simulink model "RobotSimulation1"  (R2020b)
settings: Solver=ode45  StartTime=0.0  StopTime=2  MaxStep=1e-6  RelTol=1e-3%1e-10
model workspace (MAT data in the model file):
  H = 0.2
  L = 0.1
  Mchoice = 1
  q0 = [-1.31838984174e-15; -0.785398163397; 0.0707106781187]
  qdot0 = [0; 0; 0]
settings Model: OrderedModelArguments=off  Creator=alons  LastModifiedBy=שחר צדוק
settings SolverCC: ConsecutiveZCsStepRelTol=eps%10*128*eps

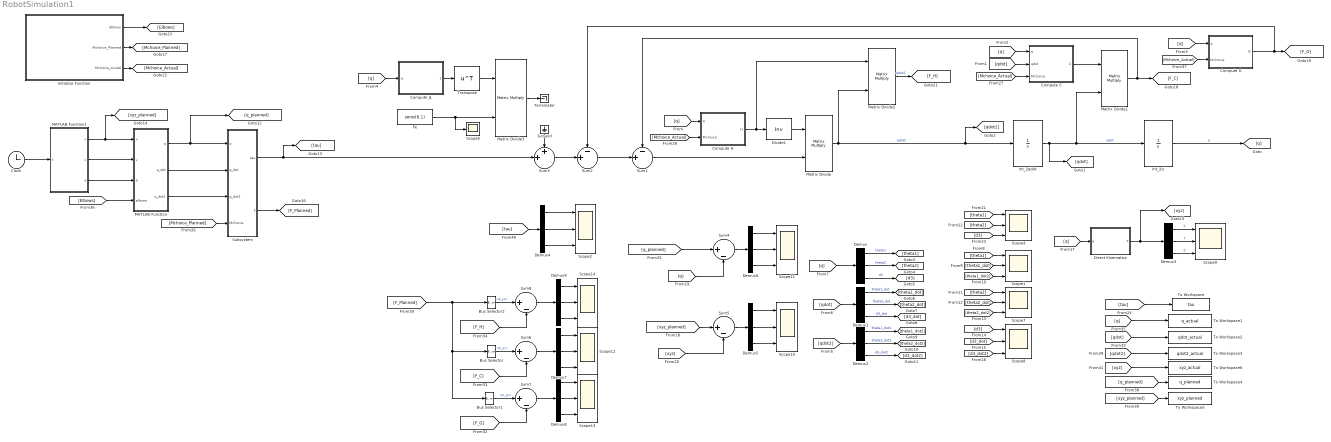
== system RobotSimulation1 ==
  Bus Selector : BusSelector  OutputSignals=F_C
  Bus Selector1 : BusSelector  OutputSignals=F_G
  Bus Selector2 : BusSelector  OutputSignals=F_H
  Clock : Clock
  Compute C : MATLAB Function  TreatAsAtomicUnit=on
  Compute G : MATLAB Function  TreatAsAtomicUnit=on
  Compute H : MATLAB Function  TreatAsAtomicUnit=on
  Compute JL : MATLAB Function  TreatAsAtomicUnit=on
  Demux{,1..9} (10 alike) : Demux  Outputs=3
  Direct Kinematics : MATLAB Function  TreatAsAtomicUnit=on
  Divide1 : Product  Inputs=/  Multiplication=Matrix(*)
  Fe : Constant  Value=zeros(6,1)
  Ground : Ground
  Initialize Function : Subsystem  TreatAsAtomicUnit=on
  Int_2q : Integrator  InitialCondition=[0,0,0]'
  Int_2qdot : Integrator  InitialCondition=[0,0,0]'
  MATLAB Function : MATLAB Function  TreatAsAtomicUnit=on
  MATLAB Function1 : MATLAB Function  TreatAsAtomicUnit=on
  Matrix Divide{,1..3} (4 alike) : Product  Inputs=**  Multiplication=Matrix(*)
  Scope{1..2,4,7..14} (11 alike) : Scope  NumInputPorts=3
  Scope5 : Scope
  Subsystem : Subsystem
  Sum1 : Sum  Inputs=-+|
  Sum2 : Sum  Inputs=-+|
  Sum3 : Sum  Inputs=++|
  Sum{4..8} (5 alike) : Sum  Inputs=|+-
  Terminator : Terminator
  To Workspace : ToWorkspace  VariableName=tau  SaveFormat=Timeseries  SampleTime=-1
  To Workspace1 : ToWorkspace  VariableName=q_actual  SaveFormat=Timeseries  SampleTime=-1
  To Workspace2 : ToWorkspace  VariableName=qdot_actual  SaveFormat=Timeseries  SampleTime=-1
  To Workspace3 : ToWorkspace  VariableName=qdot2_actual  SaveFormat=Timeseries  SampleTime=-1
  To Workspace4 : ToWorkspace  VariableName=q_planned  SaveFormat=Timeseries  SampleTime=-1
  To Workspace5 : ToWorkspace  VariableName=xyz_planned  SaveFormat=Timeseries  SampleTime=-1
  To Workspace6 : ToWorkspace  VariableName=xyz_actual  SaveFormat=Timeseries  SampleTime=-1
  Transpose : Math  Operator=transpose  SaturateOnIntegerOverflow=on
  wires:
  Compute H/1(H) -> Matrix Divide2/1, Divide1/1
  Compute C/1(C) -> Matrix Divide1/1
  Int_2qdot/1 -> [qdot], Matrix Divide1/2, Int_2q/1  "qdot"
  Int_2q/1 -> [q]  "q"
  Divide1/1 -> Matrix Divide/1
  Matrix Divide/1 -> Matrix Divide2/2, [qdot2], Int_2qdot/1  "qdot2"
  Sum2/1 -> Sum1/2
  Sum1/1 -> Matrix Divide/2
  Compute G/1(G) -> [F_G], Sum2/1
  Sum3/1 -> Sum2/2
  Compute JL/1(J) -> Transpose/1
  Transpose/1 -> Matrix Divide3/1
  Fe/1 -> Scope5/1, Matrix Divide3/2
  [q] -> Compute H/1(q)
  [qdot] -> Compute C/2(qdot)
  [q] -> Compute C/1(q)
  [q] -> Compute G/1(q)
  Matrix Divide1/1 -> [F_C], Sum1/1
  [q] -> Compute JL/1(q)
  [Mchoice_Actual] -> Compute C/3(Mchoice)
  [Mchoice_Actual] -> Compute G/2(Mchoice)
  [Mchoice_Actual] -> Compute H/2(Mchoice)
  Subsystem/1(tau) -> [tau], Sum3/2
  [q] -> Demux/1
  [qdot] -> Demux1/1
  [qdot2] -> Demux2/1
  Demux/1 -> [theta1]  "theta1"
  Demux1/1 -> [theta1_dot]  "theta1_dot"
  Demux/3 -> [d3]  "d3"
  Demux/2 -> [theta2]  "theta2"
  Demux1/2 -> [theta2_dot]  "theta2_dot"
  Demux1/3 -> [d3_dot]  "d3_dot"
  Demux2/1 -> [theta1_dot2]  "theta1_dot2"
  Demux2/2 -> [theta2_dot2]  "theta2_dot2"
  Demux2/3 -> [d3_dot2]  "d3_dot2"
  [theta1] -> Scope1/1
  [theta1_dot] -> Scope1/2
  [theta1_dot2] -> Scope1/3
  [theta2] -> Scope7/1
  [theta2_dot] -> Scope7/2
  [theta2_dot2] -> Scope7/3
  [d3] -> Scope8/1
  [d3_dot] -> Scope8/2
  [d3_dot2] -> Scope8/3
  [q] -> Direct Kinematics/1(q)
  Direct Kinematics/1(T) -> [xyz], Demux3/1
  Demux3/1 -> Scope9/1  "X"
  Demux3/2 -> Scope9/2  "Y"
  Demux3/3 -> Scope9/3  "Z"
  Demux4/1 -> Scope2/1
  Demux4/2 -> Scope2/2
  Demux4/3 -> Scope2/3
  Clock/1 -> MATLAB Function1/1(t)
  MATLAB Function1/1(x) -> [xyz_planned], MATLAB Function/1(x)
  MATLAB Function1/2(v) -> MATLAB Function/2(v)
  MATLAB Function1/3(a) -> MATLAB Function/3(a)
  [Elbows] -> MATLAB Function/4(elbows)
  MATLAB Function/2(q_dot) -> Subsystem/2(q_dot)
  MATLAB Function/3(q_dot2) -> Subsystem/3(q_dot2)
  MATLAB Function/1(q) -> [q_planned], Subsystem/1(q)
  [theta1] -> Scope4/1
  [theta2] -> Scope4/2
  [d3] -> Scope4/3
  [q_planned] -> Sum4/1
  [q] -> Sum4/2
  [xyz_planned] -> Sum5/1
  [xyz] -> Sum5/2
  Sum5/1 -> Demux5/1
  Demux5/1 -> Scope10/1
  Demux5/2 -> Scope10/2
  Demux5/3 -> Scope10/3
  Demux6/1 -> Scope11/1
  Demux6/2 -> Scope11/2
  Sum4/1 -> Demux6/1
  Demux6/3 -> Scope11/3
  [tau] -> To Workspace/1
  Subsystem/2(F) -> [F_Planned]
  [Mchoice_Planned] -> Subsystem/4(Mchoice)
  Bus Selector/1 -> Sum6/1  "<F_C>"
  [F_C] -> Sum6/2
  Sum6/1 -> Demux7/1
  Demux7/1 -> Scope12/1
  Demux7/2 -> Scope12/2
  Demux7/3 -> Scope12/3
  Bus Selector1/1 -> Sum7/1  "<F_G>"
  [F_G] -> Sum7/2
  Demux8/1 -> Scope13/1
  Demux8/2 -> Scope13/2
  Demux8/3 -> Scope13/3
  Sum7/1 -> Demux8/1
  Demux9/2 -> Scope14/2
  [F_H] -> Sum8/2
  Sum8/1 -> Demux9/1
  Demux9/3 -> Scope14/3
  Demux9/1 -> Scope14/1
  Bus Selector2/1 -> Sum8/1  "<F_H>"
  [F_Planned] -> Bus Selector1/1, Bus Selector/1, Bus Selector2/1
  Matrix Divide2/1 -> [F_H]  "qdot2"
  Initialize Function/2(Mchoice_Planned) -> [Mchoice_Planned]
  Initialize Function/1(Elbows) -> [Elbows]
  Matrix Divide3/1 -> Terminator/1
  Ground/1 -> Sum3/1
  Initialize Function/3(Mchoice_Acutal) -> [Mchoice_Actual]
  [q] -> To Workspace1/1
  [qdot] -> To Workspace2/1
  [qdot2] -> To Workspace3/1
  [xyz_planned] -> To Workspace5/1
  [q_planned] -> To Workspace4/1
  [tau] -> Demux4/1
  [xyz] -> To Workspace6/1

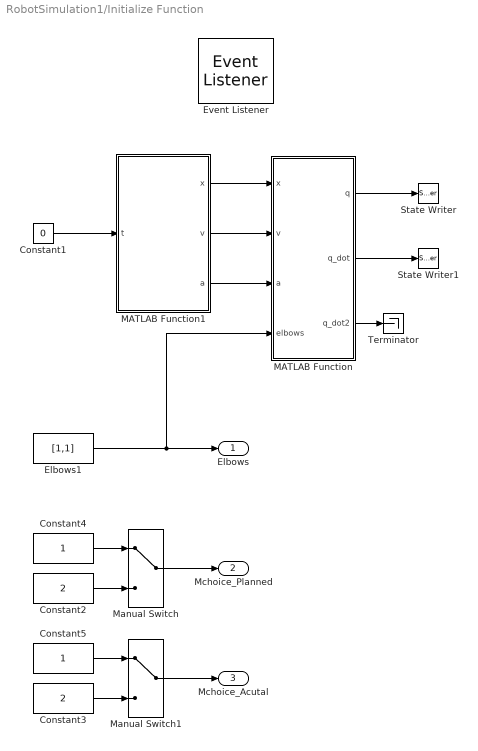
== system RobotSimulation1/Initialize Function ==
  Constant1 : Constant  Value=0
  Constant2 : Constant  Value=2
  Constant3 : Constant  Value=2
  Constant4 : Constant
  Constant5 : Constant
  Elbows1 : Constant  Value=[1,1]
  Event Listener : EventListener  DisableCoverage=on  EventName=reset
  MATLAB Function : MATLAB Function  TreatAsAtomicUnit=on
  MATLAB Function1 : MATLAB Function  TreatAsAtomicUnit=on
  Manual Switch : ManualSwitch
  Manual Switch1 : ManualSwitch
  State Writer : StateWriter  StateOwnerBlock=../../Int_2q
  State Writer1 : StateWriter  StateOwnerBlock=../../Int_2qdot
  Terminator : Terminator
  Elbows : Outport
  Mchoice_Planned : Outport  Port=2
  Mchoice_Acutal : Outport  Port=3
  wires:
  Constant1/1 -> MATLAB Function1/1(t)
  MATLAB Function1/1(x) -> MATLAB Function/1(x)
  MATLAB Function1/2(v) -> MATLAB Function/2(v)
  MATLAB Function1/3(a) -> MATLAB Function/3(a)
  Elbows1/1 -> Elbows/1, MATLAB Function/4(elbows)
  MATLAB Function/1(q) -> State Writer/1
  MATLAB Function/2(q_dot) -> State Writer1/1
  MATLAB Function/3(q_dot2) -> Terminator/1
  Constant4/1 -> Manual Switch/1
  Constant2/1 -> Manual Switch/2
  Manual Switch/1 -> Mchoice_Planned/1
  Constant3/1 -> Manual Switch1/2
  Constant5/1 -> Manual Switch1/1
  Manual Switch1/1 -> Mchoice_Acutal/1

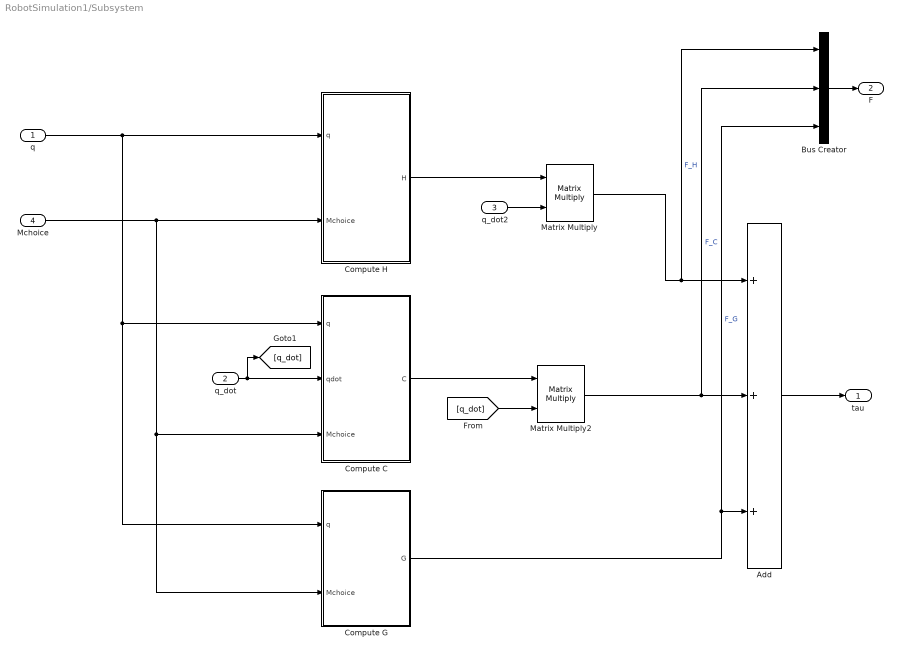
== system RobotSimulation1/Subsystem ==
  q : Inport
  q_dot : Inport  Port=2
  q_dot2 : Inport  Port=3
  Mchoice : Inport  Port=4
  Add : Sum  Inputs=+++
  Bus Creator : BusCreator  Inputs=3
  Compute C : MATLAB Function  TreatAsAtomicUnit=on
  Compute G : MATLAB Function  TreatAsAtomicUnit=on
  Compute H : MATLAB Function  TreatAsAtomicUnit=on
  Matrix Multiply : Product  Multiplication=Matrix(*)
  Matrix Multiply2 : Product  Multiplication=Matrix(*)
  tau : Outport
  F : Outport  Port=2
  wires:
  Compute H/1(H) -> Matrix Multiply/1
  Compute C/1(C) -> Matrix Multiply2/1
  q/1 -> Compute H/1(q), Compute G/1(q), Compute C/1(q)
  q_dot/1 -> Compute C/2(qdot), [q_dot]
  q_dot2/1 -> Matrix Multiply/2
  [q_dot] -> Matrix Multiply2/2
  Matrix Multiply/1 -> Bus Creator/1, Add/1  "F_H"
  Add/1 -> tau/1
  Bus Creator/1 -> F/1
  Matrix Multiply2/1 -> Bus Creator/2, Add/2  "F_C"
  Compute G/1(G) -> Bus Creator/3, Add/3  "F_G"
  Mchoice/1 -> Compute H/2(Mchoice), Compute G/2(Mchoice), Compute C/3(Mchoice)

== matlab function RobotSimulation1/Subsystem/Compute G ==
  data: q input; G output; Mchoice input
function G = ComputeG(q,Mchoice)
f_GdynM1=@(in1)[0.0;sin(in1(2,:)).*(in1(3,:).*1.0e+1-pi.*4.3875e-2+in1(3,:).*pi.*(3.51e+2./4.0e+2)).*(-4.905e-1);cos(in1(2,:)).*(pi.*4.3875e-2+1.0./2.0).*(9.81e+2./1.0e+2)];
f_GdynM2=@(in1)[0.0;sin(in1(2,:)).*(in1(3,:).*1.2e+1-pi.*4.3875e-2+in1(3,:).*pi.*(3.51e+2./4.0e+2)).*(-4.905e-1);cos(in1(2,:)).*(pi.*4.3875e-2+3.0./5.0).*(9.81e+2./1.0e+2)];
if Mchoice==1
    G=f_GdynM1(q);
else %==2
    G=f_GdynM2(q);
end
end

== matlab function RobotSimulation1/Subsystem/Compute H ==
  data: q input; H output; Mchoice input
function H = ComputeH(q,Mchoice)
f_HdynM1=@(in1)reshape([pi.*5.85e-4+(in1(3,:).^2.*sin(in1(2,:)).^2)./2.0+pi.*sin(in1(2,:)).^2.*1.4625e-4-in1(3,:).*pi.*sin(in1(2,:)).^2.*4.3875e-3+in1(3,:).^2.*pi.*sin(in1(2,:)).^2.*4.3875e-2+1.0./2.0e+2,cos(in1(2,:)).*(in1(3,:).*1.0e+1-pi.*4.3875e-2+in1(3,:).*pi.*(3.51e+2./4.0e+2)).*(-1.0./2.0e+2),sin(in1(2,:)).*(pi.*4.3875e-2+1.0./2.0).*(-1.0./1.0e+1),cos(in1(2,:)).*(in1(3,:).*1.0e+1-pi.*4.3875e-2+in1(3,:).*pi.*(3.51e+2./4.0e+2)).*(-1.0./2.0e+2),pi.*3.65625e-5+in1(3,:).^2./2.0+pi.*(in1(3,:)-1.0./2.0e+1).^2.*4.3875e-2,0.0,sin(in1(2,:)).*(pi.*4.3875e-2+1.0./2.0).*(-1.0./1.0e+1),0.0,pi.*4.3875e-2+1.0./2.0],[3,3]);
f_HdynM2=@(in1)reshape([pi.*5.85e-4+in1(3,:).^2.*sin(in1(2,:)).^2.*(3.0./5.0)+pi.*sin(in1(2,:)).^2.*1.4625e-4-in1(3,:).*pi.*sin(in1(2,:)).^2.*4.3875e-3+in1(3,:).^2.*pi.*sin(in1(2,:)).^2.*4.3875e-2+3.0./5.0e+2,cos(in1(2,:)).*(in1(3,:).*1.2e+1-pi.*4.3875e-2+in1(3,:).*pi.*(3.51e+2./4.0e+2)).*(-1.0./2.0e+2),sin(in1(2,:)).*(pi.*4.3875e-2+3.0./5.0).*(-1.0./1.0e+1),cos(in1(2,:)).*(in1(3,:).*1.2e+1-pi.*4.3875e-2+in1(3,:).*pi.*(3.51e+2./4.0e+2)).*(-1.0./2.0e+2),pi.*3.65625e-5+in1(3,:).^2.*(3.0./5.0)+pi.*(in1(3,:)-1.0./2.0e+1).^2.*4.3875e-2,0.0,sin(in1(2,:)).*(pi.*4.3875e-2+3.0./5.0).*(-1.0./1.0e+1),0.0,pi.*4.3875e-2+3.0./5.0],[3,3]);
if Mchoice==1
    H=f_HdynM1(q);
else %==2
    H=f_HdynM2(q);
end

== matlab function RobotSimulation1/Compute C ==
  data: q input; C output; qdot input; Mchoice input
function C = ComputeC(q,qdot,Mchoice)
f_CdynM1=@(in1)reshape([in1(6,:).*((in1(3,:).*sin(in1(2,:)).^2)./2.0-pi.*sin(in1(2,:)).^2.*2.19375e-3+in1(3,:).*pi.*sin(in1(2,:)).^2.*4.3875e-2)+in1(5,:).*((in1(3,:).^2.*sin(in1(2,:).*2.0))./4.0+pi.*sin(in1(2,:).*2.0).*7.3125e-5-in1(3,:).*pi.*sin(in1(2,:).*2.0).*2.19375e-3+in1(3,:).^2.*pi.*sin(in1(2,:).*2.0).*2.19375e-2),in1(4,:).*sin(in1(2,:).*2.0).*(pi.*1.755e-1-in1(3,:).*pi.*5.265+in1(3,:).^2.*pi.*5.265e+1+in1(3,:).^2.*6.0e+2).*(-4.166666666666667e-4),in1(4,:).*sin(in1(2,:)).^2.*(in1(3,:).*1.0e+1-pi.*4.3875e-2+in1(3,:).*pi.*(3.51e+2./4.0e+2)).*(-1.0./2.0e+1),in1(4,:).*((in1(3,:).^2.*sin(in1(2,:).*2.0))./4.0+pi.*sin(in1(2,:).*2.0).*7.3125e-5-in1(3,:).*pi.*sin(in1(2,:).*2.0).*2.19375e-3+in1(3,:).^2.*pi.*sin(in1(2,:).*2.0).*2.19375e-2)-in1(6,:).*((cos(in1(2,:)).*(pi.*(3.51e+2./4.0e+2)+1.0e+1))./4.0e+2+(cos(in1(2,:)).*(pi.*4.3875e-2+1.0./2.0))./2.0e+1)+(in1(5,:).*sin(in1(2,:)).*(in1(3,:).*1.0e+1-pi.*4.3875e-2+in1(3,:).*pi.*(3.51e+2./4.0e+2)))./2.0e+2,in1(6,:).*(in1(3,:)./2.0+pi.*(in1(3,:).*2.0-1.0./1.0e+1).*2.19375e-2),in1(5,:).*(in1(3,:).*1.0e+1-pi.*4.3875e-2+in1(3,:).*pi.*(3.51e+2./4.0e+2)).*(-1.0./2.0e+1),-in1(4,:).*(pi.*(cos(in1(2,:)).^2-1.0).*(-2.19375e-3)+(in1(3,:).*(cos(in1(2,:)).^2-1.0))./2.0+in1(3,:).*pi.*(cos(in1(2,:)).^2-1.0).*4.3875e-2)-in1(5,:).*((cos(in1(2,:)).*(pi.*(3.51e+2./4.0e+2)+1.0e+1))./4.0e+2+(cos(in1(2,:)).*(pi.*4.3875e-2+1.0./2.0))./2.0e+1),(in1(5,:).*(in1(3,:).*1.0e+1-pi.*4.3875e-2+in1(3,:).*pi.*(3.51e+2./4.0e+2)))./2.0e+1,0.0],[3,3]);
f_CdynM2=@(in1)reshape([in1(6,:).*(in1(3,:).*sin(in1(2,:)).^2.*(3.0./5.0)-pi.*sin(in1(2,:)).^2.*2.19375e-3+in1(3,:).*pi.*sin(in1(2,:)).^2.*4.3875e-2)+in1(5,:).*(in1(3,:).^2.*sin(in1(2,:).*2.0).*(3.0./1.0e+1)+pi.*sin(in1(2,:).*2.0).*7.3125e-5-in1(3,:).*pi.*sin(in1(2,:).*2.0).*2.19375e-3+in1(3,:).^2.*pi.*sin(in1(2,:).*2.0).*2.19375e-2),in1(4,:).*sin(in1(2,:).*2.0).*(pi.*1.755e-1-in1(3,:).*pi.*5.265+in1(3,:).^2.*pi.*5.265e+1+in1(3,:).^2.*7.2e+2).*(-4.166666666666667e-4),in1(4,:).*sin(in1(2,:)).^2.*(in1(3,:).*1.2e+1-pi.*4.3875e-2+in1(3,:).*pi.*(3.51e+2./4.0e+2)).*(-1.0./2.0e+1),in1(4,:).*(in1(3,:).^2.*sin(in1(2,:).*2.0).*(3.0./1.0e+1)+pi.*sin(in1(2,:).*2.0).*7.3125e-5-in1(3,:).*pi.*sin(in1(2,:).*2.0).*2.19375e-3+in1(3,:).^2.*pi.*sin(in1(2,:).*2.0).*2.19375e-2)-in1(6,:).*((cos(in1(2,:)).*(pi.*(3.51e+2./4.0e+2)+1.2e+1))./4.0e+2+(cos(in1(2,:)).*(pi.*4.3875e-2+3.0./5.0))./2.0e+1)+(in1(5,:).*sin(in1(2,:)).*(in1(3,:).*1.2e+1-pi.*4.3875e-2+in1(3,:).*pi.*(3.51e+2./4.0e+2)))./2.0e+2,in1(6,:).*(in1(3,:).*(3.0./5.0)+pi.*(in1(3,:).*2.0-1.0./1.0e+1).*2.19375e-2),in1(5,:).*(in1(3,:).*1.2e+1-pi.*4.3875e-2+in1(3,:).*pi.*(3.51e+2./4.0e+2)).*(-1.0./2.0e+1),-in1(4,:).*(pi.*(cos(in1(2,:)).^2-1.0).*(-2.19375e-3)+in1(3,:).*(cos(in1(2,:)).^2-1.0).*(3.0./5.0)+in1(3,:).*pi.*(cos(in1(2,:)).^2-1.0).*4.3875e-2)-in1(5,:).*((cos(in1(2,:)).*(pi.*(3.51e+2./4.0e+2)+1.2e+1))./4.0e+2+(cos(in1(2,:)).*(pi.*4.3875e-2+3.0./5.0))./2.0e+1),(in1(5,:).*(in1(3,:).*1.2e+1-pi.*4.3875e-2+in1(3,:).*pi.*(3.51e+2./4.0e+2)))./2.0e+1,0.0],[3,3]);
if Mchoice==1
    C=f_CdynM1([q;qdot]);
else %==2
    C=f_CdynM2([q;qdot]);
end
end

== matlab function RobotSimulation1/Compute H ==
  data: q input; H output; Mchoice input
function H = ComputeH(q,Mchoice)
f_HdynM1=@(in1)reshape([pi.*5.85e-4+(in1(3,:).^2.*sin(in1(2,:)).^2)./2.0+pi.*sin(in1(2,:)).^2.*1.4625e-4-in1(3,:).*pi.*sin(in1(2,:)).^2.*4.3875e-3+in1(3,:).^2.*pi.*sin(in1(2,:)).^2.*4.3875e-2+1.0./2.0e+2,cos(in1(2,:)).*(in1(3,:).*1.0e+1-pi.*4.3875e-2+in1(3,:).*pi.*(3.51e+2./4.0e+2)).*(-1.0./2.0e+2),sin(in1(2,:)).*(pi.*4.3875e-2+1.0./2.0).*(-1.0./1.0e+1),cos(in1(2,:)).*(in1(3,:).*1.0e+1-pi.*4.3875e-2+in1(3,:).*pi.*(3.51e+2./4.0e+2)).*(-1.0./2.0e+2),pi.*3.65625e-5+in1(3,:).^2./2.0+pi.*(in1(3,:)-1.0./2.0e+1).^2.*4.3875e-2,0.0,sin(in1(2,:)).*(pi.*4.3875e-2+1.0./2.0).*(-1.0./1.0e+1),0.0,pi.*4.3875e-2+1.0./2.0],[3,3]);
f_HdynM2=@(in1)reshape([pi.*5.85e-4+in1(3,:).^2.*sin(in1(2,:)).^2.*(3.0./5.0)+pi.*sin(in1(2,:)).^2.*1.4625e-4-in1(3,:).*pi.*sin(in1(2,:)).^2.*4.3875e-3+in1(3,:).^2.*pi.*sin(in1(2,:)).^2.*4.3875e-2+3.0./5.0e+2,cos(in1(2,:)).*(in1(3,:).*1.2e+1-pi.*4.3875e-2+in1(3,:).*pi.*(3.51e+2./4.0e+2)).*(-1.0./2.0e+2),sin(in1(2,:)).*(pi.*4.3875e-2+3.0./5.0).*(-1.0./1.0e+1),cos(in1(2,:)).*(in1(3,:).*1.2e+1-pi.*4.3875e-2+in1(3,:).*pi.*(3.51e+2./4.0e+2)).*(-1.0./2.0e+2),pi.*3.65625e-5+in1(3,:).^2.*(3.0./5.0)+pi.*(in1(3,:)-1.0./2.0e+1).^2.*4.3875e-2,0.0,sin(in1(2,:)).*(pi.*4.3875e-2+3.0./5.0).*(-1.0./1.0e+1),0.0,pi.*4.3875e-2+3.0./5.0],[3,3]);
if Mchoice==1
    H=f_HdynM1(q);
else %==2
    H=f_HdynM2(q);
end

== matlab function RobotSimulation1/Compute G ==
  data: q input; G output; Mchoice input
function G = ComputeG(q,Mchoice)
f_GdynM1=@(in1)[0.0;sin(in1(2,:)).*(in1(3,:).*1.0e+1-pi.*4.3875e-2+in1(3,:).*pi.*(3.51e+2./4.0e+2)).*(-4.905e-1);cos(in1(2,:)).*(pi.*4.3875e-2+1.0./2.0).*(9.81e+2./1.0e+2)];
f_GdynM2=@(in1)[0.0;sin(in1(2,:)).*(in1(3,:).*1.2e+1-pi.*4.3875e-2+in1(3,:).*pi.*(3.51e+2./4.0e+2)).*(-4.905e-1);cos(in1(2,:)).*(pi.*4.3875e-2+3.0./5.0).*(9.81e+2./1.0e+2)];
if Mchoice==1
    G=f_GdynM1(q);
else %==2
    G=f_GdynM2(q);
end
end

== matlab function RobotSimulation1/Compute JL ==
  data: q input; J output
function J = ComputeJL(q)
f_JL=@(in1)reshape([sin(in1(1,:)).*(-1.0./1.0e+1)+in1(3,:).*cos(in1(1,:)).*sin(in1(2,:)),cos(in1(1,:))./1.0e+1+in1(3,:).*sin(in1(1,:)).*sin(in1(2,:)),0.0,in1(3,:).*cos(in1(2,:)).*sin(in1(1,:)),-in1(3,:).*cos(in1(1,:)).*cos(in1(2,:)),-in1(3,:).*sin(in1(2,:)),sin(in1(1,:)).*sin(in1(2,:)),-cos(in1(1,:)).*sin(in1(2,:)),cos(in1(2,:))],[3,3]);
f_JA=@(in1)reshape([0.0,0.0,1.0,cos(in1(1,:)),sin(in1(1,:)),0.0,0.0,0.0,0.0],[3,3]);
JL=f_JL(q);
JA=f_JA(q);
J=[JL;JA];
end

== matlab function RobotSimulation1/Direct Kinematics ==
  data: T output; q input
function T = fcn(q)
f_A3t0=@(in1)reshape([cos(in1(1,:)),sin(in1(1,:)),0.0,0.0,-cos(in1(2,:)).*sin(in1(1,:)),cos(in1(1,:)).*cos(in1(2,:)),sin(in1(2,:)),0.0,sin(in1(1,:)).*sin(in1(2,:)),-cos(in1(1,:)).*sin(in1(2,:)),cos(in1(2,:)),0.0,cos(in1(1,:))./1.0e+1+in1(3,:).*sin(in1(1,:)).*sin(in1(2,:)),sin(in1(1,:))./1.0e+1-in1(3,:).*cos(in1(1,:)).*sin(in1(2,:)),in1(3,:).*cos(in1(2,:))+1.0./5.0,1.0],[4,4]);
A=f_A3t0(q);
T=A(1:3,4);
end

== matlab function RobotSimulation1/MATLAB Function ==
  data: x input; v input; a input; q output; elbows input; q_dot output; q_dot2 output
function [q,q_dot,q_dot2] = xyz2q(x,v,a,elbows)
q=inverse_kin(x,elbows);

JL=CalcJL(q);
q_dot=linsolve((JL),v);

JL_dot=CalcJLdot(q,q_dot);
q_dot2=linsolve(JL,a-JL_dot*q_dot);
end

function q=inverse_kin(x,elbows)
H=0.2;
L=0.1;

t2_elbow=elbows(1);
d3_elbow=elbows(2);
q=zeros(3,size(x,2));
for i=1:size(x,2)
    %Parse
    Px=x(1,i);
    Py=x(2,i);
    Pz=x(3,i);
    %Compute d3
    d3=d3_elbow*sqrt(Px^2+Py^2+(Pz-H)^2-L^2);
    %compute theta2
    c2=(Pz-H)/(d3+eps); %<------------Added eps
    s2=t2_elbow*sqrt(1-c2^2);
    t2=atan2(s2,c2);
    %compute theta1
    a=d3*s2;
    b=L;
    c=-Py;
    d=Px;
    t1=atan2(a*d-b*c,a*c+b*d);
    %create joint vector
    q(:,i)=[t1,t2,d3]';
end
end

function JL=CalcJL(q)
f_JL=@(in1)reshape([sin(in1(1,:)).*(-1.0./1.0e+1)+in1(3,:).*cos(in1(1,:)).*sin(in1(2,:)),cos(in1(1,:))./1.0e+1+in1(3,:).*sin(in1(1,:)).*sin(in1(2,:)),0.0,in1(3,:).*cos(in1(2,:)).*sin(in1(1,:)),-in1(3,:).*cos(in1(1,:)).*cos(in1(2,:)),-in1(3,:).*sin(in1(2,:)),sin(in1(1,:)).*sin(in1(2,:)),-cos(in1(1,:)).*sin(in1(2,:)),cos(in1(2,:))],[3,3]);
JL=f_JL(q);
end

function JLdot=CalcJLdot(q,qdot)
f_JLdot=@(in1)reshape([-in1(4,:).*(cos(in1(1,:))./1.0e+1+in1(3,:).*sin(in1(1,:)).*sin(in1(2,:)))+in1(6,:).*cos(in1(1,:)).*sin(in1(2,:))+in1(3,:).*in1(5,:).*cos(in1(1,:)).*cos(in1(2,:)),-in1(4,:).*(sin(in1(1,:))./1.0e+1-in1(3,:).*cos(in1(1,:)).*sin(in1(2,:)))+in1(6,:).*sin(in1(1,:)).*sin(in1(2,:))+in1(3,:).*in1(5,:).*cos(in1(2,:)).*sin(in1(1,:)),0.0,in1(6,:).*cos(in1(2,:)).*sin(in1(1,:))-in1(3,:).*in1(5,:).*sin(in1(1,:)).*sin(in1(2,:))+in1(3,:).*in1(4,:).*cos(in1(1,:)).*cos(in1(2,:)),-in1(6,:).*cos(in1(1,:)).*cos(in1(2,:))+in1(3,:).*in1(4,:).*cos(in1(2,:)).*sin(in1(1,:))+in1(3,:).*in1(5,:).*cos(in1(1,:)).*sin(in1(2,:)),-in1(6,:).*sin(in1(2,:))-in1(3,:).*in1(5,:).*cos(in1(2,:)),in1(4,:).*cos(in1(1,:)).*sin(in1(2,:))+in1(5,:).*cos(in1(2,:)).*sin(in1(1,:)),-in1(5,:).*cos(in1(1,:)).*cos(in1(2,:))+in1(4,:).*sin(in1(1,:)).*sin(in1(2,:)),-in1(5,:).*sin(in1(2,:))],[3,3]);
JLdot=f_JLdot([q;qdot]);
end

== matlab function RobotSimulation1/MATLAB Function1 ==
  data: t input; x output; v output; a output
function [x,v,a] = t2xyz(t)
T=2;
X0=0.1; Y0=0.05; Z0=0.25;
dX=0.15; dY=-0.2; dZ=0.1;

x=(10*(t/T)^3-15*(t/T)^4+6*(t/T)^5)*[dX,dY,dZ]'+[X0,Y0,Z0]';
v=(30*(t^2)/T^3-60*(t^3)/T^4+30*(t^4)/T^5)*[dX,dY,dZ]';
a=(60*t/T^3-180*(t^2)/T^4+120*(t^3)/T^5)*[dX,dY,dZ]';
end

== matlab function RobotSimulation1/Initialize Function/MATLAB Function1 ==
  data: t input; x output; v output; a output
function [x,v,a] = t2xyz(t)
T=2;
X0=0.1; Y0=0.05; Z0=0.25;
dX=0.15; dY=-0.2; dZ=0.1;

x=(10*(t/T)^3-15*(t/T)^4+6*(t/T)^5)*[dX,dY,dZ]'+[X0,Y0,Z0]';
v=(30*(t^2)/T^3-60*(t^3)/T^4+30*(t^4)/T^5)*[dX,dY,dZ]';
a=(60*t/T^3-180*(t^2)/T^4+120*(t^3)/T^5)*[dX,dY,dZ]';
end

== matlab function RobotSimulation1/Initialize Function/MATLAB Function ==
  data: x input; v input; a input; q output; elbows input; q_dot output; q_dot2 output
function [q,q_dot,q_dot2] = xyz2q(x,v,a,elbows)
q=inverse_kin(x,elbows);

JL=CalcJL(q);
q_dot=linsolve((JL),v);

JL_dot=CalcJLdot(q,q_dot);
q_dot2=linsolve(JL,a-JL_dot*q_dot);
end

function q=inverse_kin(x,elbows)
H=0.2;
L=0.1;

t2_elbow=elbows(1);
d3_elbow=elbows(2);
q=zeros(3,size(x,2));
for i=1:size(x,2)
    %Parse
    Px=x(1,i);
    Py=x(2,i);
    Pz=x(3,i);
    %Compute d3
    d3=d3_elbow*sqrt(Px^2+Py^2+(Pz-H)^2-L^2);
    %compute theta2
    c2=(Pz-H)/(d3+eps); %<------------Added eps
    s2=t2_elbow*sqrt(1-c2^2);
    t2=atan2(s2,c2);
    %compute theta1
    a=d3*s2;
    b=L;
    c=-Py;
    d=Px;
    t1=atan2(a*d-b*c,a*c+b*d);
    %create joint vector
    q(:,i)=[t1,t2,d3]';
end
end

function JL=CalcJL(q)
f_JL=@(in1)reshape([sin(in1(1,:)).*(-1.0./1.0e+1)+in1(3,:).*cos(in1(1,:)).*sin(in1(2,:)),cos(in1(1,:))./1.0e+1+in1(3,:).*sin(in1(1,:)).*sin(in1(2,:)),0.0,in1(3,:).*cos(in1(2,:)).*sin(in1(1,:)),-in1(3,:).*cos(in1(1,:)).*cos(in1(2,:)),-in1(3,:).*sin(in1(2,:)),sin(in1(1,:)).*sin(in1(2,:)),-cos(in1(1,:)).*sin(in1(2,:)),cos(in1(2,:))],[3,3]);
JL=f_JL(q);
end

function JLdot=CalcJLdot(q,qdot)
f_JLdot=@(in1)reshape([-in1(4,:).*(cos(in1(1,:))./1.0e+1+in1(3,:).*sin(in1(1,:)).*sin(in1(2,:)))+in1(6,:).*cos(in1(1,:)).*sin(in1(2,:))+in1(3,:).*in1(5,:).*cos(in1(1,:)).*cos(in1(2,:)),-in1(4,:).*(sin(in1(1,:))./1.0e+1-in1(3,:).*cos(in1(1,:)).*sin(in1(2,:)))+in1(6,:).*sin(in1(1,:)).*sin(in1(2,:))+in1(3,:).*in1(5,:).*cos(in1(2,:)).*sin(in1(1,:)),0.0,in1(6,:).*cos(in1(2,:)).*sin(in1(1,:))-in1(3,:).*in1(5,:).*sin(in1(1,:)).*sin(in1(2,:))+in1(3,:).*in1(4,:).*cos(in1(1,:)).*cos(in1(2,:)),-in1(6,:).*cos(in1(1,:)).*cos(in1(2,:))+in1(3,:).*in1(4,:).*cos(in1(2,:)).*sin(in1(1,:))+in1(3,:).*in1(5,:).*cos(in1(1,:)).*sin(in1(2,:)),-in1(6,:).*sin(in1(2,:))-in1(3,:).*in1(5,:).*cos(in1(2,:)),in1(4,:).*cos(in1(1,:)).*sin(in1(2,:))+in1(5,:).*cos(in1(2,:)).*sin(in1(1,:)),-in1(5,:).*cos(in1(1,:)).*cos(in1(2,:))+in1(4,:).*sin(in1(1,:)).*sin(in1(2,:)),-in1(5,:).*sin(in1(2,:))],[3,3]);
JLdot=f_JLdot([q;qdot]);
end

== matlab function RobotSimulation1/Subsystem/Compute C ==
  data: q input; C output; qdot input; Mchoice input
function C = ComputeC(q,qdot,Mchoice)
f_CdynM1=@(in1)reshape([in1(6,:).*((in1(3,:).*sin(in1(2,:)).^2)./2.0-pi.*sin(in1(2,:)).^2.*2.19375e-3+in1(3,:).*pi.*sin(in1(2,:)).^2.*4.3875e-2)+in1(5,:).*((in1(3,:).^2.*sin(in1(2,:).*2.0))./4.0+pi.*sin(in1(2,:).*2.0).*7.3125e-5-in1(3,:).*pi.*sin(in1(2,:).*2.0).*2.19375e-3+in1(3,:).^2.*pi.*sin(in1(2,:).*2.0).*2.19375e-2),in1(4,:).*sin(in1(2,:).*2.0).*(pi.*1.755e-1-in1(3,:).*pi.*5.265+in1(3,:).^2.*pi.*5.265e+1+in1(3,:).^2.*6.0e+2).*(-4.166666666666667e-4),in1(4,:).*sin(in1(2,:)).^2.*(in1(3,:).*1.0e+1-pi.*4.3875e-2+in1(3,:).*pi.*(3.51e+2./4.0e+2)).*(-1.0./2.0e+1),in1(4,:).*((in1(3,:).^2.*sin(in1(2,:).*2.0))./4.0+pi.*sin(in1(2,:).*2.0).*7.3125e-5-in1(3,:).*pi.*sin(in1(2,:).*2.0).*2.19375e-3+in1(3,:).^2.*pi.*sin(in1(2,:).*2.0).*2.19375e-2)-in1(6,:).*((cos(in1(2,:)).*(pi.*(3.51e+2./4.0e+2)+1.0e+1))./4.0e+2+(cos(in1(2,:)).*(pi.*4.3875e-2+1.0./2.0))./2.0e+1)+(in1(5,:).*sin(in1(2,:)).*(in1(3,:).*1.0e+1-pi.*4.3875e-2+in1(3,:).*pi.*(3.51e+2./4.0e+2)))./2.0e+2,in1(6,:).*(in1(3,:)./2.0+pi.*(in1(3,:).*2.0-1.0./1.0e+1).*2.19375e-2),in1(5,:).*(in1(3,:).*1.0e+1-pi.*4.3875e-2+in1(3,:).*pi.*(3.51e+2./4.0e+2)).*(-1.0./2.0e+1),-in1(4,:).*(pi.*(cos(in1(2,:)).^2-1.0).*(-2.19375e-3)+(in1(3,:).*(cos(in1(2,:)).^2-1.0))./2.0+in1(3,:).*pi.*(cos(in1(2,:)).^2-1.0).*4.3875e-2)-in1(5,:).*((cos(in1(2,:)).*(pi.*(3.51e+2./4.0e+2)+1.0e+1))./4.0e+2+(cos(in1(2,:)).*(pi.*4.3875e-2+1.0./2.0))./2.0e+1),(in1(5,:).*(in1(3,:).*1.0e+1-pi.*4.3875e-2+in1(3,:).*pi.*(3.51e+2./4.0e+2)))./2.0e+1,0.0],[3,3]);
f_CdynM2=@(in1)reshape([in1(6,:).*(in1(3,:).*sin(in1(2,:)).^2.*(3.0./5.0)-pi.*sin(in1(2,:)).^2.*2.19375e-3+in1(3,:).*pi.*sin(in1(2,:)).^2.*4.3875e-2)+in1(5,:).*(in1(3,:).^2.*sin(in1(2,:).*2.0).*(3.0./1.0e+1)+pi.*sin(in1(2,:).*2.0).*7.3125e-5-in1(3,:).*pi.*sin(in1(2,:).*2.0).*2.19375e-3+in1(3,:).^2.*pi.*sin(in1(2,:).*2.0).*2.19375e-2),in1(4,:).*sin(in1(2,:).*2.0).*(pi.*1.755e-1-in1(3,:).*pi.*5.265+in1(3,:).^2.*pi.*5.265e+1+in1(3,:).^2.*7.2e+2).*(-4.166666666666667e-4),in1(4,:).*sin(in1(2,:)).^2.*(in1(3,:).*1.2e+1-pi.*4.3875e-2+in1(3,:).*pi.*(3.51e+2./4.0e+2)).*(-1.0./2.0e+1),in1(4,:).*(in1(3,:).^2.*sin(in1(2,:).*2.0).*(3.0./1.0e+1)+pi.*sin(in1(2,:).*2.0).*7.3125e-5-in1(3,:).*pi.*sin(in1(2,:).*2.0).*2.19375e-3+in1(3,:).^2.*pi.*sin(in1(2,:).*2.0).*2.19375e-2)-in1(6,:).*((cos(in1(2,:)).*(pi.*(3.51e+2./4.0e+2)+1.2e+1))./4.0e+2+(cos(in1(2,:)).*(pi.*4.3875e-2+3.0./5.0))./2.0e+1)+(in1(5,:).*sin(in1(2,:)).*(in1(3,:).*1.2e+1-pi.*4.3875e-2+in1(3,:).*pi.*(3.51e+2./4.0e+2)))./2.0e+2,in1(6,:).*(in1(3,:).*(3.0./5.0)+pi.*(in1(3,:).*2.0-1.0./1.0e+1).*2.19375e-2),in1(5,:).*(in1(3,:).*1.2e+1-pi.*4.3875e-2+in1(3,:).*pi.*(3.51e+2./4.0e+2)).*(-1.0./2.0e+1),-in1(4,:).*(pi.*(cos(in1(2,:)).^2-1.0).*(-2.19375e-3)+in1(3,:).*(cos(in1(2,:)).^2-1.0).*(3.0./5.0)+in1(3,:).*pi.*(cos(in1(2,:)).^2-1.0).*4.3875e-2)-in1(5,:).*((cos(in1(2,:)).*(pi.*(3.51e+2./4.0e+2)+1.2e+1))./4.0e+2+(cos(in1(2,:)).*(pi.*4.3875e-2+3.0./5.0))./2.0e+1),(in1(5,:).*(in1(3,:).*1.2e+1-pi.*4.3875e-2+in1(3,:).*pi.*(3.51e+2./4.0e+2)))./2.0e+1,0.0],[3,3]);
if Mchoice==1
    C=f_CdynM1([q;qdot]);
else %==2
    C=f_CdynM2([q;qdot]);
end
end
